simulink model "md11gsnew2011"  (Simulink 7.5)
settings: Solver=ode45  StartTime=0.0  StopTime=1000  RelTol=1e-3
values from neighbouring files (symbols this model uses):
  alpha1G = 0.01    [gsnew2011.m]    (also in md11fla2011.m)
  alpha2G = 10    [gsnew2011.m]    (also in md11fla2011.m)
  alpha3G = 1    [gsnew2011.m]    (also in md11fla2011.m)
  ap = [Xu Xw 0 -g;Zu Zw Zq 0;Mu Mw Mq 0;0 0 1 0]    [gsnew2011.m]    (also in md11fla2011.m = [Xu Xw 0 -g 0;Zu Zw Zq 0 0;Mu Mw Mq 0 0;0 0 1 0 0;0 -1/U0  0)
  bp = [XL XT XR;ZL ZT ZR;ML MT MR;0 0 0]    [gsnew2011.m]    (also in md11fla2011.m = [XL XT XR;ZL ZT ZR;ML MT MR;0 0 0; 0 0 0])
  Cpg = [1 0 0 0 0 0 0;0 1/U0 0 -1 0 0 0]    [gsnew2011.m]
  gama_ref = pi/60    (= 0.0523598775598)    [gsnew2011.m]    (also in md11fla2011.m)
  GAMA_ref = 0    [gsnew2011.m]    (also in md11fla2011.m)
  h_init = 1500    [gsnew2011.m]
  Kgs1 = Kgs(:,1:7)    [gsnew2011.m]    (also in md11fla2011.m)
  Kgs2 = Kgs(:,8:10)    [gsnew2011.m]    (also in md11fla2011.m)
  ncon = 3    [gsnew2011.m]    (also in md11fla2011.m)
  np = 4    [gsnew2011.m]    (also in md11fla2011.m = 5)
  pthrot = 0.6    [gsnew2011.m]    (also in md11fla2011.m = 1)
  Rn0 = 7600    [gsnew2011.m]    (also in md11fla2011.m)
  T1 = 100    [gsnew2011.m]    (also in md11fla2011.m)
  U0 = U    (= 168.9)    [gsnew2011.m]    (also in md11fla2011.m = 295.575)
  u_ref = 0    [gsnew2011.m]    (also in md11fla2011.m = 165)
  Vc0 = 84.7    [gsnew2011.m]    (also in md11fla2011.m)
settings Model: Creator=ranjan  LastModifiedBy=knightofaccess
settings OptimizationCC: InitFltsAndDblsToZero=on
settings DebuggingCC: StrictBusMsg=Warning

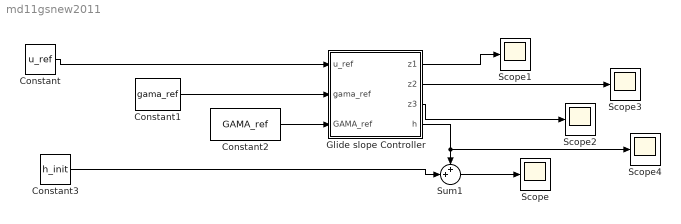
== system md11gsnew2011 ==
  Constant : Constant  Value=u_ref  OutDataType=sfix(16)  OutScaling=2^0
  Constant1 : Constant  Value=gama_ref  OutDataType=sfix(16)  OutScaling=2^0
  Constant2 : Constant  Value=GAMA_ref  OutDataType=sfix(16)  OutScaling=2^0
  Constant3 : Constant  Value=h_init  OutDataType=sfix(16)  OutScaling=2^0
  Glide slope Controller : Subsystem
  Scope{,1..4} (5 alike) : Scope
      Scope settings: YMin=-7.2e+007  YMax=-7.135e+007
      Scope2 settings: YMin=1.525e+006  YMax=1.5475e+006  SaveName=ScopeData2
      Scope3 settings: SaveName=ScopeData3
      Scope4 settings: YMin=-7.2e+007  YMax=-7.135e+007  SaveName=ScopeData4
  Sum1 : Sum  Inputs=++|  OutDataType=sfix(16)  OutScaling=2^0
  wires:
  Constant/1 -> Glide slope Controller/1(u_ref)
  Constant1/1 -> Glide slope Controller/2(gama_ref)
  Constant2/1 -> Glide slope Controller/3(GAMA_ref)
  Glide slope Controller/1(z1) -> Scope1/1
  Glide slope Controller/3(z3) -> Scope2/1
  Glide slope Controller/2(z2) -> Scope3/1
  Sum1/1 -> Scope/1
  Glide slope Controller/4(h) -> Sum1/1, Scope4/1
  Constant3/1 -> Sum1/2

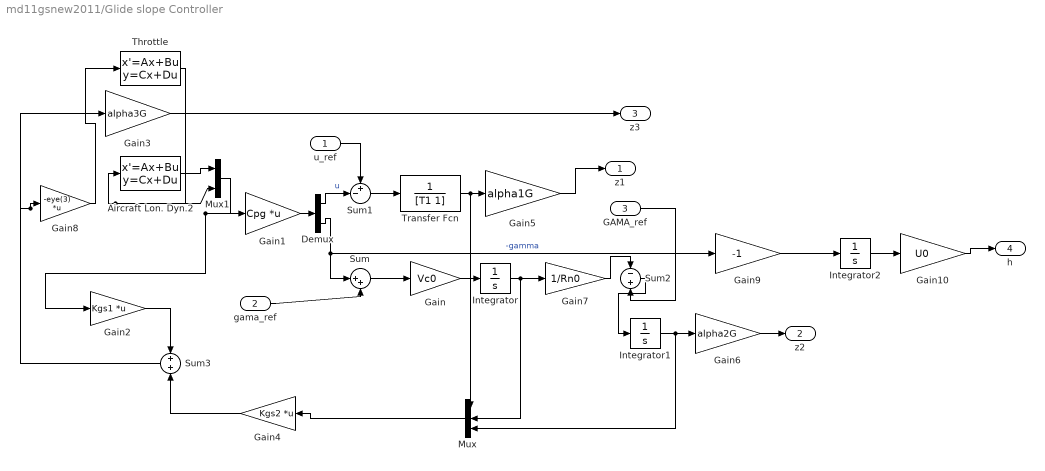
== system md11gsnew2011/Glide slope Controller ==
  u_ref : Inport  OutDataType=sfix(16)  OutScaling=2^0
  gama_ref : Inport  Port=2  OutDataType=sfix(16)  OutScaling=2^0
  GAMA_ref : Inport  Port=3  OutDataType=sfix(16)  OutScaling=2^0
  Aircraft Lon. Dyn.2 : StateSpace  A=ap  B=bp  C=eye(np)  D=zeros(np,3)
  Demux : Demux  Outputs=2
  Gain : Gain  Gain=Vc0  ParameterDataType=sfix(16)  ParameterScaling=2^0  OutDataType=sfix(16)  OutScaling=2^0
  Gain1 : Gain  Gain=Cpg  Multiplication=Matrix(K*u)  ParameterDataType=sfix(16)  ParameterScaling=2^0  OutDataType=sfix(16)  OutScaling=2^0
  Gain10 : Gain  Gain=U0  ParameterDataType=sfix(16)  ParameterScaling=2^0  OutDataType=sfix(16)  OutScaling=2^0
  Gain2 : Gain  Gain=Kgs1  Multiplication=Matrix(K*u)  ParameterDataType=sfix(16)  ParameterScaling=2^0  OutDataType=sfix(16)  OutScaling=2^0
  Gain3 : Gain  Gain=alpha3G  ParameterDataType=sfix(16)  ParameterScaling=2^0  OutDataType=sfix(16)  OutScaling=2^0
  Gain4 : Gain  Gain=Kgs2  Multiplication=Matrix(K*u)  ParameterDataType=sfix(16)  ParameterScaling=2^0  OutDataType=sfix(16)  OutScaling=2^0
  Gain5 : Gain  Gain=alpha1G  ParameterDataType=sfix(16)  ParameterScaling=2^0  OutDataType=sfix(16)  OutScaling=2^0
  Gain6 : Gain  Gain=alpha2G  ParameterDataType=sfix(16)  ParameterScaling=2^0  OutDataType=sfix(16)  OutScaling=2^0
  Gain7 : Gain  Gain=1/Rn0  ParameterDataType=sfix(16)  ParameterScaling=2^0  OutDataType=sfix(16)  OutScaling=2^0
  Gain8 : Gain  Gain=-eye(3)  Multiplication=Matrix(K*u)  ParameterDataType=sfix(16)  ParameterScaling=2^0  OutDataType=sfix(16)  OutScaling=2^0
  Gain9 : Gain  Gain=-1  ParameterDataType=sfix(16)  ParameterScaling=2^0  OutDataType=sfix(16)  OutScaling=2^0
  Integrator : Integrator
  Integrator1 : Integrator
  Integrator2 : Integrator
  Mux : Mux  Inputs=3
  Mux1 : Mux  Inputs=2
  Sum : Sum  Inputs=|++  OutDataType=sfix(16)  OutScaling=2^0
  Sum1 : Sum  Inputs=+-|  OutDataType=sfix(16)  OutScaling=2^0
  Sum2 : Sum  Inputs=-+  OutDataType=sfix(16)  OutScaling=2^0
  Sum3 : Sum  OutDataType=sfix(16)  OutScaling=2^0
  Throttle : StateSpace  A=-pthrot*eye(ncon)  B=pthrot*eye(ncon)  C=eye(3)  D=zeros(3,3)
  Transfer Fcn : TransferFcn  Denominator=[T1 1]
  z1 : Outport  OutDataType=sfix(16)  OutScaling=2^0
  z2 : Outport  Port=2  OutDataType=sfix(16)  OutScaling=2^0
  z3 : Outport  Port=3  OutDataType=sfix(16)  OutScaling=2^0
  h : Outport  Port=4  OutDataType=sfix(16)  OutScaling=2^0
  wires:
  Gain/1 -> Integrator/1
  Sum/1 -> Gain/1
  Sum1/1 -> Transfer Fcn/1
  Mux1/1 -> Gain1/1, Gain2/1
  Gain1/1 -> Demux/1
  Demux/1 -> Sum1/2  "u"
  Demux/2 -> Sum/1, Gain9/1  "-gamma"
  Gain2/1 -> Sum3/1
  Sum3/1 -> Gain3/1, Gain8/1
  Mux/1 -> Gain4/1
  Gain4/1 -> Sum3/2
  Integrator/1 -> Mux/2, Gain7/1
  Transfer Fcn/1 -> Mux/1, Gain5/1
  Gain7/1 -> Sum2/1
  Sum2/1 -> Integrator1/1
  Integrator1/1 -> Gain6/1, Mux/3
  u_ref/1 -> Sum1/1
  gama_ref/1 -> Sum/2
  GAMA_ref/1 -> Sum2/2
  Gain5/1 -> z1/1
  Gain6/1 -> z2/1
  Gain3/1 -> z3/1
  Gain9/1 -> Integrator2/1
  Integrator2/1 -> Gain10/1
  Gain10/1 -> h/1
  Throttle/1 -> Aircraft Lon. Dyn.2/1, Mux1/2
  Aircraft Lon. Dyn.2/1 -> Mux1/1
  Gain8/1 -> Throttle/1
